simulink model "Quanser_adquisicion_datos"  (R2016a)
settings: Solver=VariableStepAuto  StartTime=0.0  StopTime=1500  RelTol=1e-3
values from neighbouring files (symbols this model uses):
  tm = 0.1    [ejemplodiscretro.m]
settings Model: Creator=Daniel  LastModifiedBy=Daniel

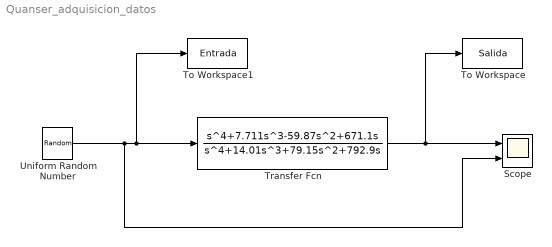
== system Quanser_adquisicion_datos ==
  Scope : Scope  NumInputPorts=2
  To Workspace : ToWorkspace  VariableName=Salida  SampleTime=tm
  To Workspace1 : ToWorkspace  VariableName=Entrada  SampleTime=tm
  Transfer Fcn : TransferFcn  Numerator=[1 7.711 -59.87 671.1 0]  Denominator=[1 14.01 79.15 792.9 0]
  Uniform Random Number : UniformRandomNumber  Minimum=0  Maximum=5  SampleTime=50
  wires:
  Transfer Fcn/1 -> Scope/1, To Workspace/1
  Uniform Random Number/1 -> Scope/2, To Workspace1/1, Transfer Fcn/1
